simulink model "Exp_03"  (R2021b)
settings: Solver=VariableStepAuto  StartTime=0.0  StopTime=10  RelTol=1e-3
libraries: slpidlib x1
settings Model: Creator=saeed  LastModifiedBy=saeed

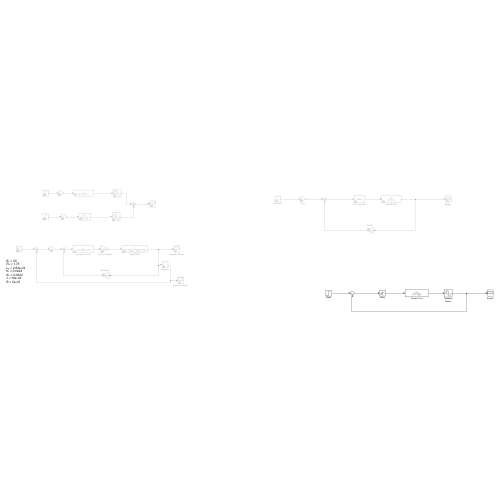
[thumbnail: Simulink's stored preview of the top-level diagram]
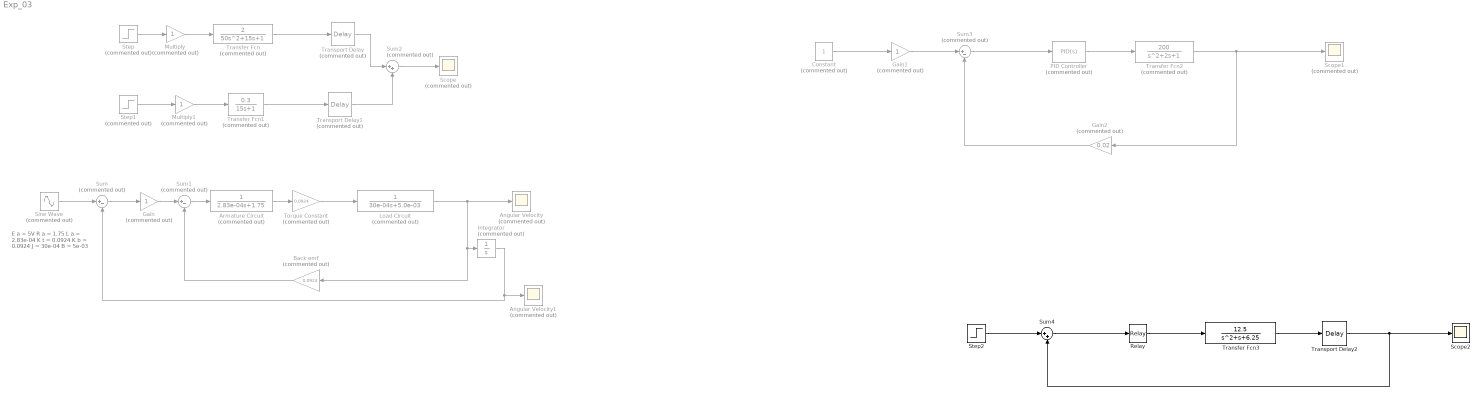
== system Exp_03 ==
  note: E a = 5V
      | R a = 1.75
      | L a = 2.83e-04
      | K t = 0.0924
      | K b = 0.0924
      | J = 30e-04
      | B = 5e-03
  Angular Velocity : Scope  Commented=on
  Angular Velocity1 : Scope  Commented=on
  Armature Circuit : TransferFcn  Commented=on  Denominator=[2.83e-04 1.75]
  Back emf : Gain  Commented=on  Gain=0.0924
  Constant : Constant  Commented=on
  Gain : Gain  Commented=on
  Gain1 : Gain  Commented=on
  Gain2 : Gain  Commented=on  Gain=0.02
  Integrator : Integrator  Commented=on
  Load Circuit : TransferFcn  Commented=on  Denominator=[30e-04 5.0e-03]
  Multiply : Gain  Commented=on
  Multiply1 : Gain  Commented=on
  PID Controller : slpidlib/PID Controller  Commented=on  Controller=PID  Form=Parallel  TimeDomain=Continuous-time  UseExternalTs=off  SampleTime=-1  IntegratorMethod=Forward Euler  FilterMethod=Forward Euler  ControllerParametersSource=internal  P=1  I=0  D=0.3  UseFilter=on  N=100  TunerSelectOption=Transfer Function Based (PID Tuner App)  InitialConditionSource=internal  InitialConditionForIntegrator=0  InitialConditionForFilter=0  DifferentiatorICPrevScaledInput=0  ExternalReset=none  TrackingMode=off  Kt=1  LimitOutput=off  SatLimitsSource=internal  UpperSaturationLimit=inf  LowerSaturationLimit=-inf  LinearizeAsGain=on  AntiWindupMode=none  Kb=1  POutMin=[]  POutMax=[]  IOutMin=[]  IOutMax=[]  DOutMin=[]  DOutMax=[]  NOutMin=[]  NOutMax=[]  SumOutMin=[]  SumOutMax=[]  SaturationOutMin=[]  SaturationOutMax=[]  PParamMin=[]  PParamMax=[]  IParamMin=[]  IParamMax=[]  DParamMin=[]  DParamMax=[]  NParamMin=[]  NParamMax=[]  KbParamMin=[]  KbParamMax=[]  KtParamMin=[]  KtParamMax=[]  KbOutMin=[]  KbOutMax=[]  KtOutMin=[]  KtOutMax=[]  IntegratorOutMin=[]  IntegratorOutMax=[]  FilterOutMin=[]  FilterOutMax=[]  SumI1OutMin=[]  SumI1OutMax=[]  SumI2OutMin=[]  SumI2OutMax=[]  SumI3OutMin=[]  SumI3OutMax=[]  SumI4OutMin=[]  SumI4OutMax=[]  SumDOutMin=[]  SumDOutMax=[]  DifferentiatorOutMin=[]  DifferentiatorOutMax=[]  FilterDiffOutCoefMin=[]  FilterDiffOutCoefMax=[]  ReciprocalOutMin=[]  ReciprocalOutMax=[]  SumDenOutMin=[]  SumDenOutMax=[]  SumNumOutMin=[]  SumNumOutMax=[]  DivideOutMin=[]  DivideOutMax=[]  UdiffTsProdOutMin=[]  UdiffTsProdOutMax=[]  NTsProdOutMin=[]  NTsProdOutMax=[]  UintegralTsProdOutMin=[]  UintegralTsProdOutMax=[]  UngainTsProdOutMin=[]  UngainTsProdOutMax=[]  IntegratorContinuousStateAttributes=''  IntegratorStateMustResolveToSignalObject=off  IntegratorRTWStateStorageClass=Auto  FilterContinuousStateAttributes=''  FilterStateMustResolveToSignalObject=off  FilterRTWStateStorageClass=Auto  ParallelPVariant=InternalParameters  IdealPVariant=Disabled  IVariant=InternalParameters  DVariant=InternalParameters  IntegratorVariant=Continuous  SatVariant=Disabled  AWVariant=Passthrough  PCopyVariant=Disabled  TRVariant=Disabled  FdbkBlocksVariant=Forward  IdealPFdbkVariant=Disabled  SatFdbkVariant=Disabled  DerivativeFilterVariant=ContFilter  NVariant=InternalParameters  NCopyVariant=Disabled  FilterICVariant=InternalICsFilter  IntegratorICVariant=InternalICs  ExternalResetVariant=Disabled  TRSumVariant=Passthrough  SumFdbkVariant=Disabled  SumVariant=Sum_PID  TsampFilterVariant=InternalTs  TsampNgainVariant=Passthrough  TsampIntegralVariant=Passthrough  ExternalSaturationOutDataTypeStr=Inherit: Same as second input
  Relay : Relay
  Scope : Scope  Commented=on
  Scope1 : Scope  Commented=on
  Scope2 : Scope
  Sine Wave : Sin  Commented=on  SampleTime=0
  Step : Step  Commented=on  SampleTime=0
  Step1 : Step  Commented=on  SampleTime=0
  Step2 : Step  SampleTime=0
  Sum : Sum  Commented=on  Inputs=|+-
  Sum1 : Sum  Commented=on  Inputs=|+-
  Sum2 : Sum  Commented=on  Inputs=|++
  Sum3 : Sum  Commented=on  Inputs=|+-
  Sum4 : Sum  Inputs=|++
  Torque Constant : Gain  Commented=on  Gain=0.0924
  Transfer Fcn : TransferFcn  Commented=on  Numerator=[2]  Denominator=[50 15 1]
  Transfer Fcn1 : TransferFcn  Commented=on  Numerator=[0.3]  Denominator=[15 1]
  Transfer Fcn2 : TransferFcn  Commented=on  Numerator=[200]
  Transfer Fcn3 : TransferFcn  Numerator=[12.5]  Denominator=[1 1 6.25]
  Transport Delay : TransportDelay  Commented=on  DelayTime=5
  Transport Delay1 : TransportDelay  Commented=on  DelayTime=5
  Transport Delay2 : TransportDelay  DelayTime=5
  wires:
  Sum/1 -> Gain/1
  Armature Circuit/1 -> Torque Constant/1
  Torque Constant/1 -> Load Circuit/1
  Load Circuit/1 -> Back emf/1, Integrator/1, Angular Velocity/1
  Integrator/1 -> Sum/2, Angular Velocity1/1
  Back emf/1 -> Sum1/2
  Sum1/1 -> Armature Circuit/1
  Gain/1 -> Sum1/1
  Sine Wave/1 -> Sum/1
  Step1/1 -> Multiply1/1
  Step/1 -> Multiply/1
  Multiply/1 -> Transfer Fcn/1
  Multiply1/1 -> Transfer Fcn1/1
  Transfer Fcn/1 -> Transport Delay/1
  Transfer Fcn1/1 -> Transport Delay1/1
  Transport Delay/1 -> Sum2/1
  Transport Delay1/1 -> Sum2/2
  Sum2/1 -> Scope/1
  Constant/1 -> Gain1/1
  Gain1/1 -> Sum3/1
  Sum3/1 -> PID Controller/1
  PID Controller/1 -> Transfer Fcn2/1
  Transfer Fcn2/1 -> Gain2/1, Scope1/1
  Gain2/1 -> Sum3/2
  Step2/1 -> Sum4/1
  Sum4/1 -> Relay/1
  Relay/1 -> Transfer Fcn3/1
  Transfer Fcn3/1 -> Transport Delay2/1
  Transport Delay2/1 -> Sum4/2, Scope2/1
